simulink model "PMSG2"  (Simulink 8.1)
settings: Solver=ode45  StartTime=0.0  StopTime=14  RelTol=1e-3
libraries: neural x1, simulink x1
settings Model: Creator=korichi  LastModifiedBy=apple
settings OptimizationCC: InitFltsAndDblsToZero=on
settings DebuggingCC: StrictBusMsg=Warning

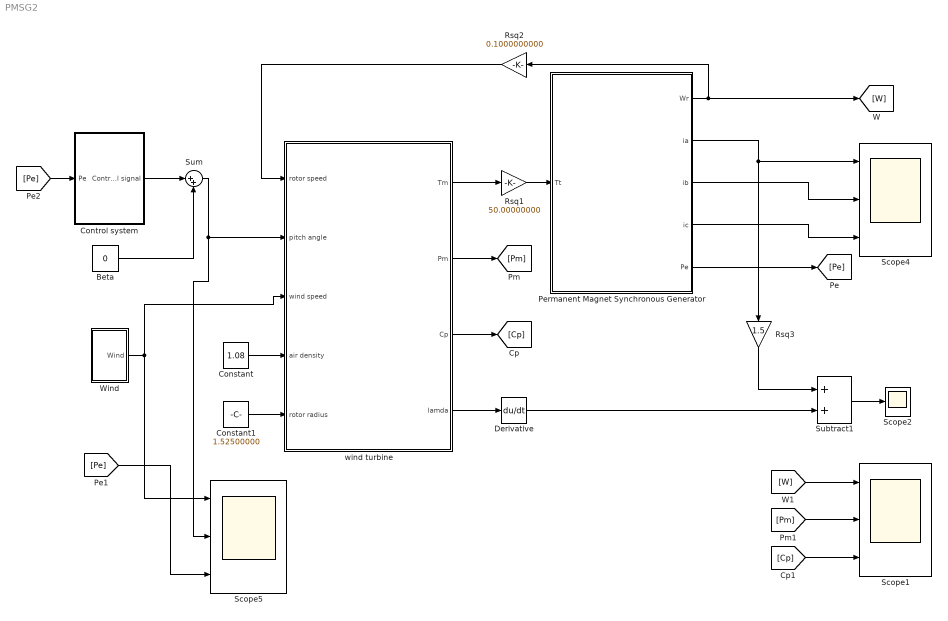
== system PMSG2 ==
  Beta : Constant  Value=0
  Constant : Constant  Value=1.08
  Constant1 : Constant  Value=1.52500000
  Control system : Subsystem
  Derivative : Derivative
  Permanent Magnet Synchronous Generator : Subsystem
  Rsq1 : Gain  Gain=50.00000000
  Rsq2 : Gain  Gain=0.1000000000
  Rsq3 : Gain  Gain=1.5
  Scope1 : Scope  NumInputPorts=3
      settings: YMin=44.7~25.25~0.0187  YMax=46.3~27.75~0.0205  SaveName=TeW2  MaxDataPoints=100000000
  Scope2 : Scope
      settings: TimeRange=10  YMin=-9  YMax=9  SaveName=TeW  MaxDataPoints=100000000  SampleInput=on
  Scope4 : Scope  NumInputPorts=3
      settings: YMin=-0.7~-0.7~-0.7  YMax=0.7~0.7~0.7  SaveName=TeW6  MaxDataPoints=100000000
  Scope5 : Scope  NumInputPorts=3
      settings: TimeRange=10  YMin=4~35~0  YMax=8~87.5~14  SaveName=TeW7  MaxDataPoints=100000000  SampleInput=on
  Subtract1 : Sum
  Sum : Sum  Inputs=|++
  Wind : Subsystem
  wind turbine : Subsystem
  wires:
  Constant/1 -> wind turbine/4(air density)
  Constant1/1 -> wind turbine/5(rotor radius)
  wind turbine/1(Tm) -> Rsq1/1
  Rsq2/1 -> wind turbine/1(rotor speed)
  Rsq1/1 -> Permanent Magnet Synchronous Generator/1(Tt)
  wind turbine/3(Cp) -> [Cp]
  wind turbine/2(Pm) -> [Pm]
  [Cp] -> Scope1/3
  [Pm] -> Scope1/2
  [W] -> Scope1/1
  Permanent Magnet Synchronous Generator/2(ia) -> Scope4/1, Rsq3/1
  Rsq3/1 -> Subtract1/1
  wind turbine/4(lamda) -> Derivative/1
  Derivative/1 -> Subtract1/2
  Permanent Magnet Synchronous Generator/1(Wr) -> [W], Rsq2/1
  Subtract1/1 -> Scope2/1
  Permanent Magnet Synchronous Generator/3(ib) -> Scope4/2
  Permanent Magnet Synchronous Generator/4(ic) -> Scope4/3
  Wind/1(Wind) -> Scope5/1, wind turbine/3(wind speed)
  Permanent Magnet Synchronous Generator/5(Pe) -> [Pe]
  Beta/1 -> Sum/2
  Sum/1 -> wind turbine/2(pitch angle), Scope5/2
  [Pe] -> Scope5/3
  [Pe] -> Control system/1(Pe)
  Control system/1(Control signal) -> Sum/1

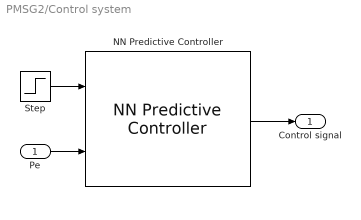
== system PMSG2/Control system ==
  Pe : Inport
  NN Predictive Controller : neural/Control Systems/NN Predictive Controller  epochs=200  minp=3.2140510716770598  maxp=87.353350358455415  mint=-0.0046658159735702065  maxt=87.353350358455415  Normalize=0  IW=[-51.792699443231825 55.073390883772454;-35.117797280370461 34.951580792286649;5.364237235495497 -3.7519058812995167;1.2837742420912039 -0.79845690049355289;2.561574732132041 1.5813855298462558;20.669038605124108 -20.671330178787628;4.1187499540259642 7.5003293024765618;15.216202633730774 -15.415087334861193;2.7889715038606018 -0.78408257484300059;-26.42378757461967 26.455910240956577;-16.282009555589827 16.711299624844191;112.9282238109827 -6.6208606685511828;13.828589507058352 13.703974301820507;-8.3733774143861073 0.22835293535077961;-14.029443333715983 -19.428471263646166;-0.43104843119523095 -0.48706196890699299;-10.430033566987989 14.860986125459956;13.28310123435462 -11.251542881426817;-52.701711785789136 -27.821479398658138;-1.2421271622957026 3.305698430750923]  LW1_2=[-91.362372862785762 83.153460333942306;16.631215283543249 -14.048399643587551;-24.823258245154403 23.846419441294028;5.0618808112857918 -7.0979340449435755;2.5829230091745368 -0.82236624948062231;-0.26634250298115847 0.10241179289510548;2.6071396488702301 1.987251442670235;2.2050563291414558 -1.4901141956615707;-36.471664282373887 25.160802507050121;0.05708128426808215 -0.089183563311683575;-6.4511859290928504 -0.31190931218952866;-4.9829557104457578 -3.7264379894110675;18.757257380459411 16.140799355056515;6.2802017259183351 -0.096949936637894613;-4.1516101104115188 2.8628866249481666;-0.70509052740305955 -0.067773840126055862;-7.1441763326552969 5.3038578372855438;-20.592266171616345 9.4575954633602084;-4.4993085343580503 -4.3379571080611328;-1.8640641877929891 2.2609767764968134]  LW2_1=[0.43350012554553596 -0.040334175531919897 0.59989239259320859 -0.018494269399628477 0.35066225018397934 -6.2981964304071809 1.5467408752053635 1.2678707783940881 0.36476237222330765 -4.5907358498443669 -1.5380349242308862 -0.35423854176607439 4.4440591061830119 -0.22456088268531654 -0.52944329559383951 -0.35426658775603248 1.5982570961095213 0.57633685846652472 -2.2519523211509473 -1.3891398263369843]  B1=[73.569796172217821;-5.871379882162195;-78.284106321967172;-2.9850603944468932;0.39641491179864435;2.0365628878961393;-1.6677244268563389;3.0257982854058367;14.214539860064876;0.77614040844869625;-7.1122649167208731;-3.2678908582097783;4.3774331807869888;12.228586072021765;-1.3492119107852321;-1.196875644024187;-5.0552226852037023;15.36627611835368;1.7575595596160856;-16.658395964648477]  B2=5.1588801144815495  max_i_int=15  min_i_int=2  limit_output=1  max_output=16  min_output=0  Use_Previous_Weights=1  N2=7  Nu=2  Ts=0.2  rho=0.05  alpha=0.001  csrchfun=csrchbac  maxiter=2  S1=20  Ni=2  Nj=2  sim_file=PMSG_PLANE  trainfun=trainlm  Use_validation=1  Use_Testing=0  max_i=90  min_i=0  sam_training=200
  Step : Step  After=15  SampleTime=0
  Control signal : Outport
  wires:
  Step/1 -> NN Predictive Controller/1
  Pe/1 -> NN Predictive Controller/2
  NN Predictive Controller/1 -> Control signal/1

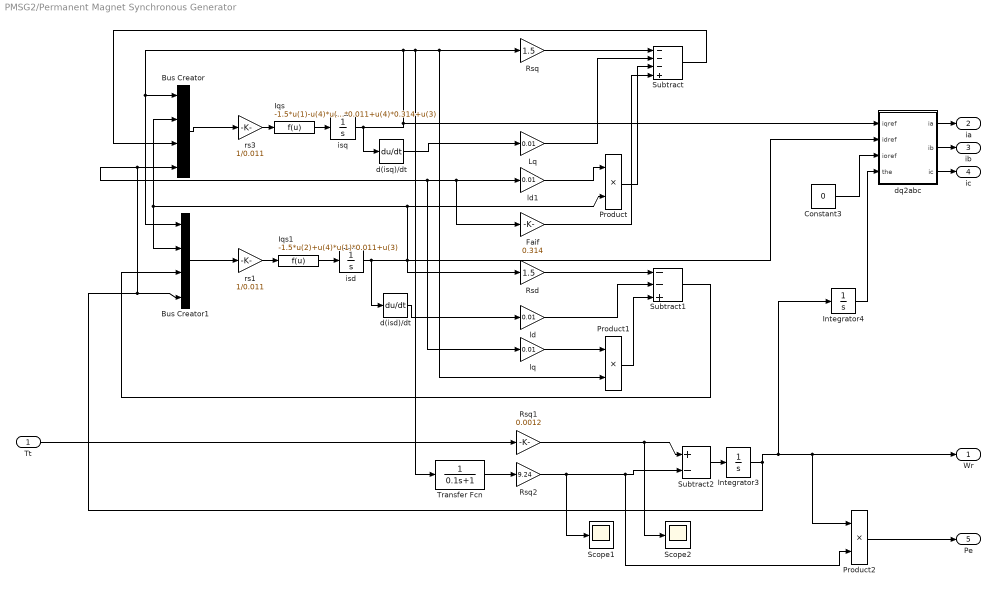
== system PMSG2/Permanent Magnet Synchronous Generator ==
  Tt : Inport
  Bus Creator : BusCreator
  Bus Creator1 : BusCreator
  Constant3 : Constant  Value=0
  Faif : Gain  Gain=0.314
  Integrator3 : Integrator  InitialCondition=1  IgnoreLimit=on
  Integrator4 : Integrator
  Iqs : Fcn  Expr=-1.5*u(1)-u(4)*u(2)*0.011+u(4)*0.314+u(3)
  Iqs1 : Fcn  Expr=-1.5*u(2)+u(4)*u(1)*0.011+u(3)
  Lq : Gain  Gain=0.01
  Product : Product  RndMeth=Zero
  Product1 : Product  RndMeth=Zero
  Product2 : Product  RndMeth=Zero
  Rsd : Gain  Gain=1.5
  Rsq : Gain  Gain=1.5
  Rsq1 : Gain  Gain=0.0012
  Rsq2 : Gain  Gain=9.24
  Scope1 : Scope
      settings: TimeRange=10  YMin=0.65  YMax=1.4  SaveName=TeW5  MaxDataPoints=100000000  SampleInput=on
  Scope2 : Scope
      settings: TimeRange=10  YMin=-30  YMax=15  SaveName=TeW4  MaxDataPoints=100000000  SampleInput=on
  Subtract : Sum  Inputs=---+
  Subtract1 : Sum  Inputs=--+
  Subtract2 : Sum  Inputs=+-
  Transfer Fcn : TransferFcn  Denominator=[0.1 1]
  d(isd)/dt : Derivative
  d(isq)/dt : Derivative
  dq2abc : Subsystem
  isd : Integrator
  isq : Integrator
  ld : Gain  Gain=0.01
  ld1 : Gain  Gain=0.01
  lq : Gain  Gain=0.01
  rs1 : Gain  Gain=1/0.011
  rs3 : Gain  Gain=1/0.011
  Wr : Outport
  ia : Outport  Port=2
  ib : Outport  Port=3
  ic : Outport  Port=4
  Pe : Outport  Port=5
  wires:
  Rsq/1 -> Subtract/1
  Iqs/1 -> isq/1
  rs3/1 -> Iqs/1
  Bus Creator/1 -> rs3/1
  Rsq1/1 -> Scope2/1, Subtract2/1
  Rsq2/1 -> Scope1/1, Product2/2, Subtract2/2
  Subtract2/1 -> Integrator3/1
  Iqs1/1 -> isd/1
  rs1/1 -> Iqs1/1
  Bus Creator1/1 -> rs1/1
  Constant3/1 -> dq2abc/3(ioref)
  dq2abc/1(ia) -> ia/1
  isq/1 -> Bus Creator/1, Bus Creator1/1, Transfer Fcn/1, Product1/2, Rsq/1, dq2abc/1(iqref), d(isq)/dt/1
  isd/1 -> Bus Creator/2, Bus Creator1/2, Product/2, dq2abc/2(idref), Rsd/1, d(isd)/dt/1
  Lq/1 -> Subtract/2
  ld1/1 -> Product/1
  Product/1 -> Subtract/3
  Faif/1 -> Subtract/4
  Rsd/1 -> Subtract1/1
  ld/1 -> Subtract1/2
  Subtract/1 -> Bus Creator/3
  lq/1 -> Product1/1
  Product1/1 -> Subtract1/3
  Subtract1/1 -> Bus Creator1/3
  Tt/1 -> Rsq1/1
  Integrator3/1 -> Wr/1, Product2/1, Integrator4/1, Bus Creator1/4, Bus Creator/4, ld1/1, Faif/1, lq/1
  d(isq)/dt/1 -> Lq/1
  d(isd)/dt/1 -> ld/1
  Integrator4/1 -> dq2abc/4(the)
  dq2abc/2(ib) -> ib/1
  dq2abc/3(ic) -> ic/1
  Product2/1 -> Pe/1
  Transfer Fcn/1 -> Rsq2/1

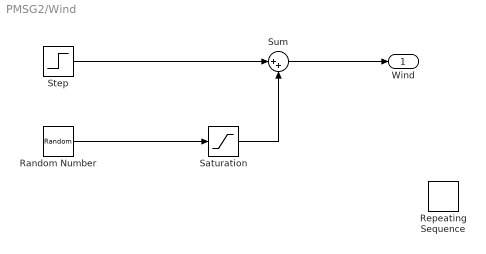
== system PMSG2/Wind ==
  Random Number : RandomNumber  Seed=20  SampleTime=0
  Repeating Sequence : simulink/Sources/Repeating Sequence  rep_seq_t=[0 2]  rep_seq_y=[0 2]
  Saturation : Saturate  UpperLimit=12  LowerLimit=5
  Step : Step  After=2  SampleTime=0
  Sum : Sum  Inputs=|++
  Wind : Outport
  wires:
  Random Number/1 -> Saturation/1
  Saturation/1 -> Sum/2
  Sum/1 -> Wind/1
  Step/1 -> Sum/1

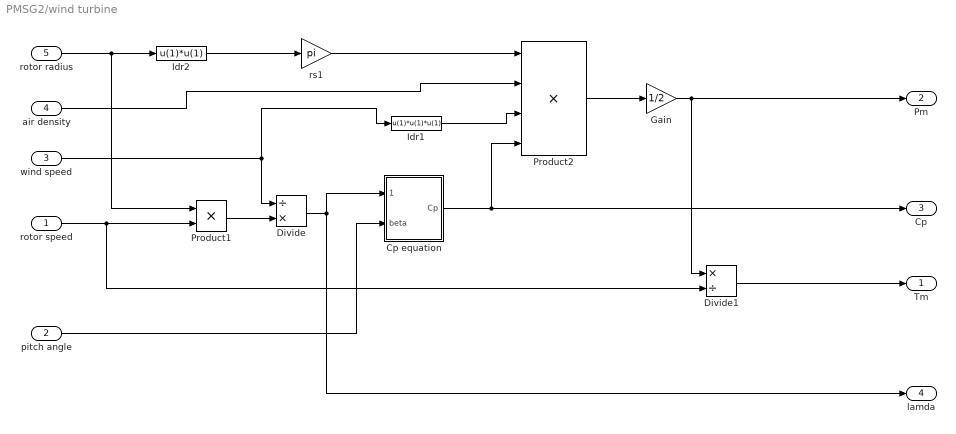
== system PMSG2/wind turbine ==
  rotor speed : Inport
  pitch angle : Inport  Port=2
  wind speed : Inport  Port=3
  air density : Inport  Port=4
  rotor radius : Inport  Port=5
  Cp equation : Subsystem
  Divide : Product  Inputs=/*
  Divide1 : Product  Inputs=*/
  Gain : Gain  Gain=1/2
  Idr1 : Fcn  Expr=u(1)*u(1)*u(1)
  Idr2 : Fcn  Expr=u(1)*u(1)
  Product1 : Product  RndMeth=Zero
  Product2 : Product  Inputs=4  RndMeth=Zero
  rs1 : Gain  Gain=pi
  Tm : Outport
  Pm : Outport  Port=2
  Cp : Outport  Port=3
  lamda : Outport  Port=4
  wires:
  Cp equation/1(Cp) -> Product2/4, Cp/1
  Divide/1 -> Cp equation/1(lambda), lamda/1
  rotor speed/1 -> Product1/2, Divide1/2
  Gain/1 -> Divide1/1, Pm/1
  air density/1 -> Product2/2
  Idr1/1 -> Product2/3
  Product2/1 -> Gain/1
  rotor radius/1 -> Product1/1, Idr2/1
  wind speed/1 -> Idr1/1, Divide/1
  Product1/1 -> Divide/2
  rs1/1 -> Product2/1
  Idr2/1 -> rs1/1
  Divide1/1 -> Tm/1
  pitch angle/1 -> Cp equation/2(beta)

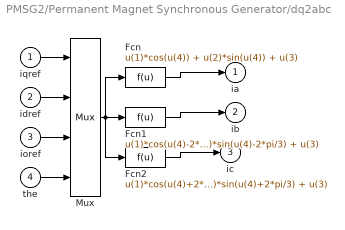
== system PMSG2/Permanent Magnet Synchronous Generator/dq2abc ==
  iqref : Inport
  idref : Inport  Port=2
  ioref : Inport  Port=3
  the : Inport  Port=4
  Fcn : Fcn  Expr=u(1)*cos(u(4)) + u(2)*sin(u(4)) + u(3)
  Fcn1 : Fcn  Expr=u(1)*cos(u(4)-2*pi/3) + u(2)*sin(u(4)-2*pi/3) + u(3)
  Fcn2 : Fcn  Expr=u(1)*cos(u(4)+2*pi/3)+ u(2)*sin(u(4)+2*pi/3) + u(3)
  Mux : Mux
  ia : Outport  InitialOutput=0
  ib : Outport  Port=2  InitialOutput=0
  ic : Outport  Port=3  InitialOutput=0
  wires:
  the/1 -> Mux/4
  ioref/1 -> Mux/3
  idref/1 -> Mux/2
  iqref/1 -> Mux/1
  Mux/1 -> Fcn1/1, Fcn2/1, Fcn/1
  Fcn1/1 -> ib/1
  Fcn/1 -> ia/1
  Fcn2/1 -> ic/1

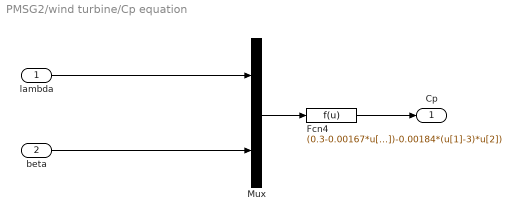
== system PMSG2/wind turbine/Cp equation ==
  lambda : Inport
  beta : Inport  Port=2
  Fcn4 : Fcn  Expr=(0.3-0.00167*u[2])*sin(pi*(u[1]+0.1)/(10-0.3*u[2])-0.00184*(u[1]-3)*u[2])
  Mux : Mux  Inputs=2
  Cp : Outport
  wires:
  beta/1 -> Mux/2
  lambda/1 -> Mux/1
  Fcn4/1 -> Cp/1
  Mux/1 -> Fcn4/1
